simulink model "KalmanandPid"  (Simulink 7.9)
settings: Solver=ode3  StartTime=0.0  StopTime=10  FixedStep=0.0004  RelTol=1e-3
undefined symbols (not defined in the file): dfilt, ObserveKalmanpid
libraries: simulink x1, dsparch4 x1
settings Model: Creator=紫盛  LastModifiedBy=紫盛

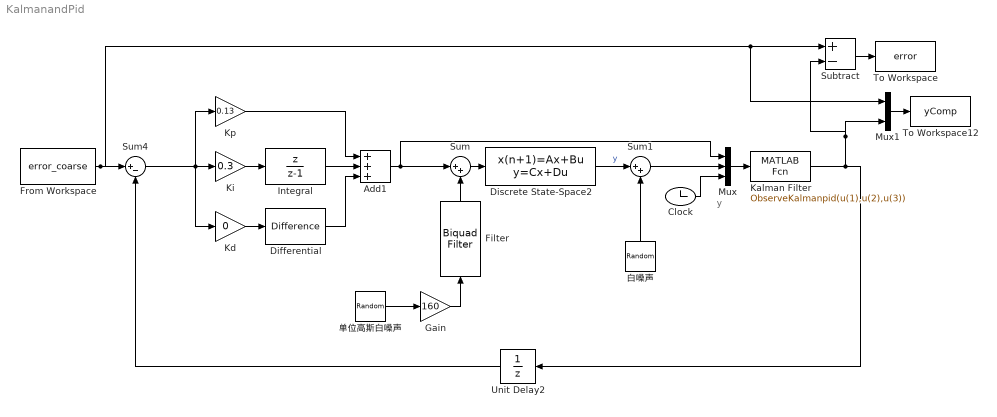
== system KalmanandPid ==
  note: y
  Add1 : Sum  Inputs=+++
  Clock : Clock
  Differential : simulink/Discrete/Difference  ICPrevInput=0.0  InputProcessing=Inherited  OutMin=[]  OutMax=[]  OutDataType=fixdt(1, 16)  OutScaling=2^-10  DoSatur=off
  Discrete State-Space2 : DiscreteStateSpace  A=[0 1;-0.005117 -0.1288]  B=[0;1]  C=[0.1 1.034]  D=[0]  SampleTime=0.0004
  Filter : dsparch4/Biquad Filter  Tag=BlockMethodSubSystem  IIRFiltStruct=Direct form II  CoeffSource=Specify via dialog  BiQuadCoeffs=[1 2 1 1 -1.99413763811177 0.994154771607242]  a0Flag=Warning  IC=0  ICnum=0  ICden=0  InputProcessing=Columns as channels (frame based)  denAccumFracLength=30  denProdOutputFracLength=30  secondMemoryFracLength=15  roundingMode=Floor  overflowMode=off  ScaleValues=[4.28337386700199e-06;1]  optimizeScaleValues=on  ScaleValueMode=Specify via input port (g)  scaleValueFracLength=14  FilterSource=Specify via dialog  dfiltObjectName=dfilt.df2tsos([1 0.3 0.4],[1 0.1 0.2])
  From Workspace : FromWorkspace  VariableName=error_coarse  SampleTime=0.0004
  Gain : Gain  Gain=160
  Integral : DiscreteTransferFcn  Numerator=[1 0]  Denominator=[1 -1]
  Kalman Filter : MATLABFcn  MATLABFcn=ObserveKalmanpid(u(1),u(2),u(3))  OutputDimensions=1
  Kd : Gain  Gain=0
  Ki : Gain  Gain=0.3
  Kp : Gain  Gain=0.13
  Mux : Mux  Inputs=3
  Mux1 : Mux  Inputs=2
  Subtract : Sum  Inputs=+-
  Sum : Sum  Inputs=|++
  Sum1 : Sum  Inputs=|++
  Sum4 : Sum  Inputs=|+-
  To Workspace : ToWorkspace  VariableName=error  SampleTime=-1  SaveFormat=Timeseries
  To Workspace12 : ToWorkspace  VariableName=yComp  SampleTime=-1  SaveFormat=Timeseries
  Unit Delay2 : UnitDelay  SampleTime=0.0004
  单位高斯白噪声 : RandomNumber  SampleTime=0.0004
  白噪声 : RandomNumber  Variance=6.5  SampleTime=0.0004
  wires:
  Mux/1 -> Kalman Filter/1
  Sum/1 -> Discrete State-Space2/1
  Discrete State-Space2/1 -> Sum1/1  "y"
  Sum1/1 -> Mux/2
  Kalman Filter/1 -> Subtract/2, Mux1/2, Unit Delay2/1
  Subtract/1 -> To Workspace/1
  Add1/1 -> Sum/1, Mux/1
  Gain/1 -> Filter/1
  单位高斯白噪声/1 -> Gain/1
  Ki/1 -> Integral/1
  Kd/1 -> Differential/1
  Kp/1 -> Add1/1
  Integral/1 -> Add1/2
  Differential/1 -> Add1/3
  Clock/1 -> Mux/3
  Filter/1 -> Sum/2
  Sum4/1 -> Ki/1, Kp/1, Kd/1
  From Workspace/1 -> Sum4/1, Subtract/1, Mux1/1
  Mux1/1 -> To Workspace12/1
  Unit Delay2/1 -> Sum4/2
  白噪声/1 -> Sum1/2
